simulink model "Simulation_Series"  (R2025b)
settings: Solver=VariableStepAuto  StartTime=0.0  StopTime=30000  RelTol=1e-6  EnableMultiTasking=on
PreLoadFcn:
  | % 1. Get the absolute path of the folder where this Simulink model is saved
  | model_dir = fileparts(get_param(bdroot, 'FileName'));
  | 
  | % 2. Add that folder and all subfolders (optimization, gp_models) to the MATLAB path
  | addpath(genpath(model_dir));
  | 
  | % 3. Print a success message to the Command Window so the user knows it worked
  | disp(['[RTO Setup] Successfully loaded paths for model: ', bdroot]);
InitFcn:
  | X_init_series
values from neighbouring files (symbols this model uses):
  Xinit1 = [          95322.9245471678 ... (first row only)    [X_init_series.m]
  Xinit2 = [139339.471687902 ... (first row only)    [X_init_series.m]
libraries: slpidlib x2, simulink x1
settings Model: Creator=chmemer  LastModifiedBy=ld719
settings SolverCC: AlgebraicLoopSolver=TrustRegion
settings DataIOCC: LimitDataPoints=on  SaveFinalState=on  SaveFormat=Array  SignalLoggingSaveFormat=ModelDataLogs  ReturnWorkspaceOutputs=off
settings OptimizationCC: ExpressionDepthLimit=2147483647.0  LifeSpan=inf
settings DebuggingCC: UnderspecifiedInitializationDetection=Classic  MergeDetectMultiDrivingBlocksExec=none  SolverPrmCheckMsg=warning  FcnCallInpInsideContextMsg=warning  UnconnectedInputMsg=warning  UnconnectedOutputMsg=warning  UnconnectedLineMsg=warning  StateNameClashWarn=warning  SFUnexpectedBacktrackingDiag=warning  SFNoUnconditionalDefaultTransitionDiag=warning  SFExecutionAtInitializationDiag=none  ArithmeticOperatorsInVariantConditions=warning
settings HardwareCC: ProdBitPerPointer=32.0  ProdBitPerSizeT=32.0  ProdBitPerPtrDiffT=32.0  ProdLargestAtomicFloat=None  ProdIntDivRoundTo=Undefined  ProdEndianess=Unspecified  ProdWordSize=32.0  ProdHWDeviceType=32-bit Generic
settings ModelReferenceCC: EnableRefExpFcnMdlSchedulingChecks=on  PropagateSignalLabelsOutOfModel=off
settings SFSimCC: SimUseLocalCustomCode=off  CustomCodeUndefinedFunction=UseInterfaceOnly
settings RTWCC: RTWUseLocalCustomCode=off  GPUComputeCapability=3.5
settings CodeAppCC: StateflowObjectComments=on
settings GRTTargetCC: TargetLangStandard=C89/C90 (ANSI)  CombineOutputUpdateFcns=off  GRTInterface=on
settings ConfigComp: CovMetricSettings=dw  CovSaveCumulativeToWorkspaceVar=on  CovSaveSingleToWorkspaceVar=on  CovExternalEMLEnable=off  CovSFcnEnable=off

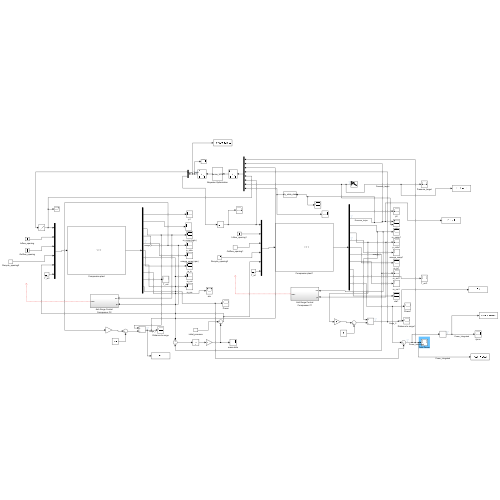
[thumbnail: Simulink's stored preview of the top-level diagram]
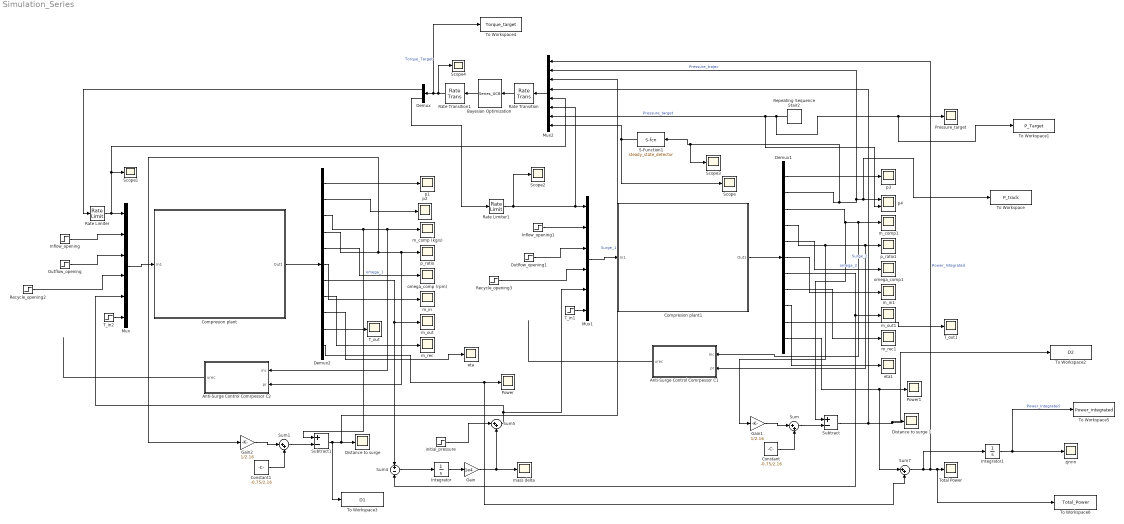
== system Simulation_Series ==
  Anti-Surge Control Comrpessor C1 : Subsystem
  Anti-Surge Control Comrpessor C2 : Subsystem
  Bayesian Optimization : S-Function  FunctionName=Series_UCB  SFunctionDeploymentMode=off  EnableBusSupport=off
  Compresion plant : Subsystem
      mask Display: image(imread('comp_plant.jpg'))
  Compresion plant1 : Subsystem
      mask Display: image(imread('comp_plant.jpg'))
  Constant : Constant  Value=-0.75/2.16
  Constant1 : Constant  Value=-0.75/2.16
  Demux : Demux  Outputs=2
  Demux1 : Demux  Outputs=11
  Demux2 : Demux  Outputs=11
  Distance to surge : Scope
      settings: ActiveDisplayYMinimum=0.077548735618170245  ActiveDisplayYMaximum=0.26199999787444433  DataLoggingVariableName=ScopeData2
  Distance to surge 1 : Scope
      settings: ActiveDisplayYMinimum=-0.020292289353042135  ActiveDisplayYMaximum=0.33961238201814714
  Gain : Gain  Gain=1e4
  Gain1 : Gain  Gain=1/2.16
  Gain2 : Gain  Gain=1/2.16
  Inflow_opening : Step  Time=25  Before=0.5  After=0.5  SampleTime=0
  Inflow_opening1 : Step  Time=25  Before=0.4541  After=0.4541  SampleTime=0
  Integrator : Integrator
  Integrator1 : Integrator
  Mux : Mux  Inputs=6
  Mux1 : Mux  Inputs=6
  Mux2 : Mux  Inputs=8
  Outflow_opening : Step  Time=10  Before=0.46  After=0.46  SampleTime=0
  Outflow_opening1 : Step  Time=10  Before=0.56  After=0.56  SampleTime=0
  Power : Scope
      settings: ActiveDisplayYMinimum=100000  ActiveDisplayYMaximum=300000  DataLoggingVariableName=ScopeData3  DataLoggingSaveFormat=Array
  Power1 : Scope
      settings: ActiveDisplayYMinimum=30000  ActiveDisplayYMaximum=70000  DataLoggingVariableName=ScopeData4  DataLoggingSaveFormat=Array
  Pressure_target : Scope
      settings: ActiveDisplayYMinimum=-1  ActiveDisplayYMaximum=1  DataLoggingVariableName=ScopeData5
  Rate Limiter : RateLimiter  RisingSlewLimit=0.1  FallingSlewLimit=-0.1  SampleTimeMode=inherited
  Rate Limiter1 : RateLimiter  RisingSlewLimit=0.1  FallingSlewLimit=-0.1  SampleTimeMode=inherited
  Rate Transition : RateTransition
  Rate Transition1 : RateTransition  InitialCondition=[20;20]
  Recycle_opening2 : Step  Time=2.05  After=0  SampleTime=0
  Recycle_opening3 : Step  Time=2.05  After=0  SampleTime=0
  Repeating Sequence Stair2 : simulink/Sources/Repeating Sequence Stair  OutValues=[248000 244000 246000 243000 242000 241000].'  tsamp=5000  OutMin=[]  OutMax=[]  OutDataTypeStr=double  OutputDataTypeScalingMode=double  OutDataType=fixdt(0,8)  ConRadixGroup=Best Precision: Vector-wise  OutScaling=2^-12
  S-Function1 : S-Function  FunctionName=steady_state_detector  SFunctionDeploymentMode=off  EnableBusSupport=off
  Scope{,1..4} (5 alike) : Scope
      Scope settings: ActiveDisplayYMinimum=-0.12499999999999997  ActiveDisplayYMaximum=1.125
      Scope1 settings: ActiveDisplayYMinimum=12.704969172625178  ActiveDisplayYMaximum=20.810558980819426  DataLoggingVariableName=ScopeData2
      Scope2 settings: ActiveDisplayYMinimum=14.056047000321247  ActiveDisplayYMaximum=20.660439222186529  DataLoggingVariableName=ScopeData3
      Scope3 settings: ActiveDisplayYMinimum=240000  ActiveDisplayYMaximum=250000
      Scope4 settings: ActiveDisplayYMinimum=10.651075634209118  ActiveDisplayYMaximum=21.457913073387115
  Subtract : Sum  Inputs=+-
  Subtract1 : Sum  Inputs=+-
  Sum{,1,5,7} (4 alike) : Sum  Inputs=|++
  Sum4 : Sum  Inputs=+|-
  T_in1 : Step  Time=2  Before=273+20  After=273+20  SampleTime=0
  T_in2 : Step  Time=2  Before=273+20  After=273+20  SampleTime=0
  T_out : Scope
      settings: ActiveDisplayYMinimum=-1  ActiveDisplayYMaximum=1
  T_out1 : Scope
      settings: ActiveDisplayYMinimum=97544.29295  ActiveDisplayYMaximum=97745.86123  DataLoggingVariableName=ScopeData2
  To Workspace : ToWorkspace  VariableName=P_track  SaveFormat=Structure With Time  SampleTime=1
  To Workspace1 : ToWorkspace  VariableName=P_Target  SaveFormat=Structure With Time  SampleTime=1
  To Workspace2 : ToWorkspace  VariableName=D2  SaveFormat=Structure With Time  SampleTime=1
  To Workspace3 : ToWorkspace  VariableName=D1  SaveFormat=Structure With Time  SampleTime=1
  To Workspace4 : ToWorkspace  VariableName=Torque_target  SaveFormat=Structure With Time  SampleTime=1
  To Workspace5 : ToWorkspace  VariableName=Power_integrated  SaveFormat=Structure With Time  SampleTime=1
  To Workspace6 : ToWorkspace  VariableName=Total_Power  SaveFormat=Structure With Time  SampleTime=1
  Total Power : Scope
      settings: ActiveDisplayYMinimum=87673.50775599209  ActiveDisplayYMaximum=243371.1571212415  DataLoggingVariableName=ScopeData3
  eta : Scope
      settings: ActiveDisplayYMinimum=0.21745085276170312  ActiveDisplayYMaximum=0.23352090021491981  DataLoggingSaveFormat=Array
  eta1 : Scope
      settings: ActiveDisplayYMinimum=0.84842072953292291  ActiveDisplayYMaximum=0.8942963809934541  DataLoggingVariableName=ScopeData2  DataLoggingSaveFormat=Array
  initial_pressure : Step  Time=30  Before=148276.78289724  After=148276.78289724  SampleTime=0
  m_comp (kg/s) : Scope
      settings: ActiveDisplayYMinimum=0.40770202444342352  ActiveDisplayYMaximum=0.84430507901595309  DataLoggingVariableName=m_comp  DataLoggingSaveFormat=Array
  m_comp1 : Scope
      settings: ActiveDisplayYMinimum=0.60292  ActiveDisplayYMaximum=0.60459  DataLoggingVariableName=m_comp1  DataLoggingSaveFormat=Array
  m_in : Scope
      settings: ActiveDisplayYMinimum=0.60226  ActiveDisplayYMaximum=0.61057  DataLoggingVariableName=ScopeData2
  m_in1 : Scope
      settings: DataLoggingVariableName=ScopeData11
  m_out : Scope
      settings: ActiveDisplayYMinimum=0.42270198893071659  ActiveDisplayYMaximum=0.77722336304535555  DataLoggingVariableName=ScopeData3
  m_out1 : Scope
      settings: ActiveDisplayYMinimum=0.50120300179820743  ActiveDisplayYMaximum=0.71721824106829912  DataLoggingVariableName=ScopeData13
  m_rec : Scope
      settings: ActiveDisplayYMinimum=-1  ActiveDisplayYMaximum=1  DataLoggingVariableName=m_rec  DataLoggingSaveFormat=Array
  m_rec1 : Scope
      settings: ActiveDisplayYMinimum=-1  ActiveDisplayYMaximum=1  DataLoggingVariableName=m_rec1  DataLoggingSaveFormat=Array
  mass delta : Scope
      settings: ActiveDisplayYMinimum=-1573.08764  ActiveDisplayYMaximum=14157.77212
  omega_comp (rpm) : Scope
      settings: TimeSpan=10  ActiveDisplayYMinimum=3418.211911212803  ActiveDisplayYMaximum=3418.2119165301274  DataLoggingVariableName=ScopeData4
  omega_comp1 : Scope
      settings: TimeSpan=10  ActiveDisplayYMinimum=3403.3405459456822  ActiveDisplayYMaximum=4015.4960771962442  DataLoggingVariableName=ScopeData14
  p1 : Scope
      settings: ActiveDisplayYMinimum=96759.18199  ActiveDisplayYMaximum=106424.4061
  p2 : Scope
      settings: TimeSpan=800  ActiveDisplayYMinimum=142686.83533455073  ActiveDisplayYMaximum=177417.85344844157
  p3 : Scope
      settings: ActiveDisplayYMinimum=129412.56133  ActiveDisplayYMaximum=141037.29748  DataLoggingVariableName=ScopeData15
  p4 : Scope  NumInputPorts=2
      settings: TimeSpan=16000  ActiveDisplayYMinimum=240988.04397616221  ActiveDisplayYMaximum=249610.22414713461  DataLoggingVariableName=ScopeData16
  p_ratio : Scope
      settings: ActiveDisplayYMinimum=1.4510137511633545  ActiveDisplayYMaximum=1.8639764896836617  DataLoggingVariableName=p_ratio  DataLoggingSaveFormat=Array
  p_ratio1 : Scope
      settings: ActiveDisplayYMinimum=1.7222858302327289  ActiveDisplayYMaximum=2.0157667356513191  DataLoggingVariableName=p_ratio1  DataLoggingSaveFormat=Array
  zjnnn : Scope
      settings: ActiveDisplayYMinimum=-2.475946022057547E+8  ActiveDisplayYMaximum=2.2283514198517928E+9
  wires:
  Compresion plant/1(Out1) -> Demux2/1
  Mux/1 -> Compresion plant/1(In1)
  Demux2/3 -> Anti-Surge Control Comrpessor C2/1(mc), m_comp (kg/s)/1, Subtract1/1
  Demux2/4 -> Gain2/1, p_ratio/1, Anti-Surge Control Comrpessor C2/2(pr)
  Demux2/5 -> omega_comp (rpm)/1  "omega_1"
  Outflow_opening/1 -> Mux/3
  Anti-Surge Control Comrpessor C2/1(urec) -> ?
  Demux2/6 -> m_in/1
  Demux2/1 -> p1/1
  Demux2/2 -> p2/1
  Demux2/8 -> m_rec/1
  Demux1/8 -> m_rec1/1
  Demux1/1 -> p3/1
  Demux1/7 -> Sum4/2, m_out1/1
  Demux1/6 -> m_in1/1
  Anti-Surge Control Comrpessor C1/1(urec) -> ?
  Outflow_opening1/1 -> Mux1/3
  Demux1/5 -> omega_comp1/1  "omega_2"
  Demux1/4 -> Gain1/1, Anti-Surge Control Comrpessor C1/2(pr), p_ratio1/1
  Demux1/3 -> Subtract/1, Anti-Surge Control Comrpessor C1/1(mc), m_comp1/1
  Mux1/1 -> Compresion plant1/1(In1)
  Compresion plant1/1(Out1) -> Demux1/1
  Sum4/1 -> Integrator/1
  Integrator/1 -> Gain/1
  initial_pressure/1 -> Sum5/1
  Sum5/1 -> Mux/5, Mux1/5
  Gain/1 -> Sum5/2, mass delta/1
  Demux2/9 -> eta/1
  Demux2/11 -> Sum7/2, Power/1
  Demux2/10 -> T_out/1
  Inflow_opening/1 -> Mux/2
  Demux1/9 -> eta1/1
  Demux1/11 -> Sum7/1, Power1/1
  T_in2/1 -> Mux/6
  Inflow_opening1/1 -> Mux1/2
  T_in1/1 -> Mux1/6
  Demux1/10 -> T_out1/1
  Integrator1/1 -> To Workspace5/1, zjnnn/1  "Power_Integrated"
  Demux2/7 -> m_out/1, Sum4/1
  Gain1/1 -> Sum/1
  Constant/1 -> Sum/2
  Sum/1 -> Subtract/2
  Subtract/1 -> Mux2/4, To Workspace2/1, Distance to surge 1/1  "Surge_2"
  Constant1/1 -> Sum1/2
  Sum1/1 -> Subtract1/2
  Gain2/1 -> Sum1/1
  Subtract1/1 -> Distance to surge/1, Mux2/3, To Workspace3/1  "Surge_1"
  Repeating Sequence Stair2/1 -> To Workspace1/1, Pressure_target/1, p4/2, Mux2/7  "Pressure_target"
  S-Function1/1 -> Mux2/8, Scope/1
  Mux2/1 -> Rate Transition/1
  Bayesian Optimization/1 -> Rate Transition1/1
  Demux1/2 -> Scope3/1, S-Function1/1, Mux2/2, To Workspace/1, p4/1  "Pressure_trajec"
  Rate Limiter1/1 -> Scope2/1, Mux2/6, Mux1/1
  Rate Limiter/1 -> Scope1/1, Mux2/5, Mux/1
  Rate Transition/1 -> Bayesian Optimization/1
  Rate Transition1/1 -> Scope4/1, To Workspace4/1, Demux/1  "Torque_Target"
  Demux/2 -> Rate Limiter1/1
  Demux/1 -> Rate Limiter/1
  Sum7/1 -> Integrator1/1, To Workspace6/1, Total Power/1, Mux2/1  "Power_Integrated"
  Recycle_opening2/1 -> Mux/4
  Recycle_opening3/1 -> Mux1/4

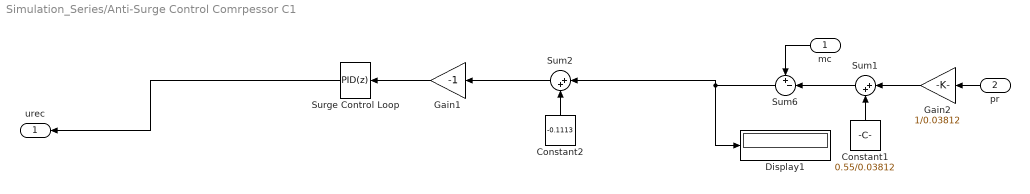
== system Simulation_Series/Anti-Surge Control Comrpessor C1 ==
  mc : Inport
  pr : Inport  Port=2
  Constant1 : Constant  Value=0.55/0.03812
  Constant2 : Constant  Value=-0.1113
  Display1 : Display
  Gain1 : Gain  Gain=-1
  Gain2 : Gain  Gain=1/0.03812
  Sum1 : Sum  Inputs=|++
  Sum2 : Sum  Inputs=|++
  Sum6 : Sum  Inputs=+-|
  Surge Control Loop : slpidlib/PID Controller  Controller=PID  Form=Parallel  TimeDomain=Discrete-time  UseExternalTs=off  SampleTime=0.5  IntegratorMethod=Forward Euler  FilterMethod=Forward Euler  ControllerParametersSource=internal  P=0.05  I=0.01  UseKiTs=off  D=0  UseExternalDerivativeSource=off  N=2.82959055969234  UseFilter=on  TunerSelectOption=Transfer Function Based (PID Tuner App)  ZeroCross=off  InitialConditionSource=internal  InitialConditionForIntegrator=0  InitialConditionForFilter=0  DifferentiatorICPrevScaledInput=0  ExternalReset=none  TrackingMode=off  Kt=1  LimitOutput=on  SatLimitsSource=internal  UpperSaturationLimit=1  LowerSaturationLimit=0  LinearizeAsGain=off  AntiWindupMode=back-calculation  Kb=1  LimitIntegrator=off  UpperIntegratorSaturationLimit=inf  LowerIntegratorSaturationLimit=-inf  POutMin=[]  POutMax=[]  IOutMin=[]  IOutMax=[]  DOutMin=[]  DOutMax=[]  NOutMin=[]  NOutMax=[]  SumOutMin=[]  SumOutMax=[]  SaturationOutMin=[]  SaturationOutMax=[]  PParamMin=[]  PParamMax=[]  IParamMin=[]  IParamMax=[]  DParamMin=[]  DParamMax=[]  NParamMin=[]  NParamMax=[]  KbParamMin=[]  KbParamMax=[]  KtParamMin=[]  KtParamMax=[]  KbOutMin=[]  KbOutMax=[]  KtOutMin=[]  KtOutMax=[]  IntegratorOutMin=[]  IntegratorOutMax=[]  FilterOutMin=[]  FilterOutMax=[]  SumI1OutMin=[]  SumI1OutMax=[]  SumI2OutMin=[]  SumI2OutMax=[]  SumI3OutMin=[]  SumI3OutMax=[]  SumI4OutMin=[]  SumI4OutMax=[]  SumDOutMin=[]  SumDOutMax=[]  DifferentiatorOutMin=[]  DifferentiatorOutMax=[]  FilterDiffOutCoefMin=[]  FilterDiffOutCoefMax=[]  ReciprocalOutMin=[]  ReciprocalOutMax=[]  SumDenOutMin=[]  SumDenOutMax=[]  SumNumOutMin=[]  SumNumOutMax=[]  DivideOutMin=[]  DivideOutMax=[]  UdiffTsProdOutMin=[]  UdiffTsProdOutMax=[]  NTsProdOutMin=[]  NTsProdOutMax=[]  UintegralTsProdOutMin=[]  UintegralTsProdOutMax=[]  UngainTsProdOutMin=[]  UngainTsProdOutMax=[]  ClampingZeroOutDataTypeStr=Inherit: Inherit via back propagation  ClampingZeroOutMin=[]  ClampingZeroOutMax=[]  FilterDenConstantOutDataTypeStr=Inherit: Inherit via back propagation  FilterDenConstantOutMin=[]  FilterDenConstantOutMax=[]  PCopyOutDataTypeStr=Inherit: Inherit via back propagation  PCopyOutMin=[]  PCopyOutMax=[]  NCopyOutDataTypeStr=Inherit: Inherit via back propagation  NCopyOutMin=[]  NCopyOutMax=[]  IntegratorContinuousStateAttributes=''  IntegratorStateMustResolveToSignalObject=off  IntegratorRTWStateStorageClass=Auto  FilterContinuousStateAttributes=''  FilterStateMustResolveToSignalObject=off  FilterRTWStateStorageClass=Auto  ParallelPVariant=InternalParameters  IdealPVariant=Disabled  IVariant=InternalParameters  DVariant=InternalParameters  IntegratorVariant=Discrete  SatVariant=Enabled  AWVariant=BackCalculation  PCopyVariant=Disabled  TRVariant=Disabled  FdbkBlocksVariant=Forward  IdealPFdbkVariant=Disabled  SatFdbkVariant=Disabled  DerivativeFilterVariant=ForwardEulerFilter  NVariant=InternalParameters  NCopyVariant=Disabled  FilterICVariant=InternalICsFilter  IntegratorICVariant=InternalICs  ExternalResetVariant=Disabled  TRSumVariant=Passthrough  SumFdbkVariant=Disabled  SumVariant=Sum_PID  TsampFilterVariant=InternalTs  TsampNgainVariant=Passthrough  TsampIntegralVariant=Disabled_SignalSpec  ExternalSaturationOutDataTypeStr=Inherit: Same as second input  DerivativeSourceVariant=ErrorSignal  PreIntVariant=InternalPreInt
  urec : Outport
  wires:
  Gain2/1 -> Sum1/1
  Constant1/1 -> Sum1/2
  Sum1/1 -> Sum6/2
  Sum6/1 -> Sum2/1, Display1/1
  Surge Control Loop/1 -> urec/1
  mc/1 -> Sum6/1
  pr/1 -> Gain2/1
  Gain1/1 -> Surge Control Loop/1
  Sum2/1 -> Gain1/1
  Constant2/1 -> Sum2/2

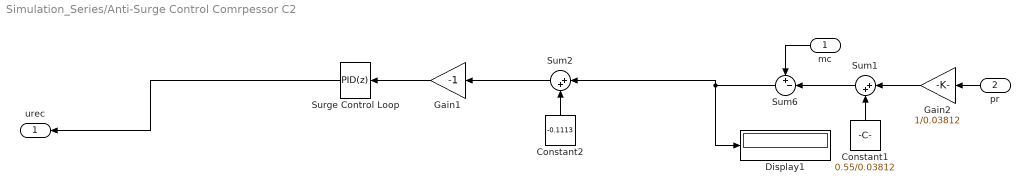
== system Simulation_Series/Anti-Surge Control Comrpessor C2 ==
  mc : Inport
  pr : Inport  Port=2
  Constant1 : Constant  Value=0.55/0.03812
  Constant2 : Constant  Value=-0.1113
  Display1 : Display
  Gain1 : Gain  Gain=-1
  Gain2 : Gain  Gain=1/0.03812
  Sum1 : Sum  Inputs=|++
  Sum2 : Sum  Inputs=|++
  Sum6 : Sum  Inputs=+-|
  Surge Control Loop : slpidlib/PID Controller  Controller=PID  Form=Parallel  TimeDomain=Discrete-time  UseExternalTs=off  SampleTime=0.5  IntegratorMethod=Forward Euler  FilterMethod=Forward Euler  ControllerParametersSource=internal  P=0.05  I=0.01  UseKiTs=off  D=0  UseExternalDerivativeSource=off  N=2.82959055969234  UseFilter=on  TunerSelectOption=Transfer Function Based (PID Tuner App)  ZeroCross=off  InitialConditionSource=internal  InitialConditionForIntegrator=0  InitialConditionForFilter=0  DifferentiatorICPrevScaledInput=0  ExternalReset=none  TrackingMode=off  Kt=1  LimitOutput=on  SatLimitsSource=internal  UpperSaturationLimit=1  LowerSaturationLimit=0  LinearizeAsGain=off  AntiWindupMode=back-calculation  Kb=1  LimitIntegrator=off  UpperIntegratorSaturationLimit=inf  LowerIntegratorSaturationLimit=-inf  POutMin=[]  POutMax=[]  IOutMin=[]  IOutMax=[]  DOutMin=[]  DOutMax=[]  NOutMin=[]  NOutMax=[]  SumOutMin=[]  SumOutMax=[]  SaturationOutMin=[]  SaturationOutMax=[]  PParamMin=[]  PParamMax=[]  IParamMin=[]  IParamMax=[]  DParamMin=[]  DParamMax=[]  NParamMin=[]  NParamMax=[]  KbParamMin=[]  KbParamMax=[]  KtParamMin=[]  KtParamMax=[]  KbOutMin=[]  KbOutMax=[]  KtOutMin=[]  KtOutMax=[]  IntegratorOutMin=[]  IntegratorOutMax=[]  FilterOutMin=[]  FilterOutMax=[]  SumI1OutMin=[]  SumI1OutMax=[]  SumI2OutMin=[]  SumI2OutMax=[]  SumI3OutMin=[]  SumI3OutMax=[]  SumI4OutMin=[]  SumI4OutMax=[]  SumDOutMin=[]  SumDOutMax=[]  DifferentiatorOutMin=[]  DifferentiatorOutMax=[]  FilterDiffOutCoefMin=[]  FilterDiffOutCoefMax=[]  ReciprocalOutMin=[]  ReciprocalOutMax=[]  SumDenOutMin=[]  SumDenOutMax=[]  SumNumOutMin=[]  SumNumOutMax=[]  DivideOutMin=[]  DivideOutMax=[]  UdiffTsProdOutMin=[]  UdiffTsProdOutMax=[]  NTsProdOutMin=[]  NTsProdOutMax=[]  UintegralTsProdOutMin=[]  UintegralTsProdOutMax=[]  UngainTsProdOutMin=[]  UngainTsProdOutMax=[]  ClampingZeroOutDataTypeStr=Inherit: Inherit via back propagation  ClampingZeroOutMin=[]  ClampingZeroOutMax=[]  FilterDenConstantOutDataTypeStr=Inherit: Inherit via back propagation  FilterDenConstantOutMin=[]  FilterDenConstantOutMax=[]  PCopyOutDataTypeStr=Inherit: Inherit via back propagation  PCopyOutMin=[]  PCopyOutMax=[]  NCopyOutDataTypeStr=Inherit: Inherit via back propagation  NCopyOutMin=[]  NCopyOutMax=[]  IntegratorContinuousStateAttributes=''  IntegratorStateMustResolveToSignalObject=off  IntegratorRTWStateStorageClass=Auto  FilterContinuousStateAttributes=''  FilterStateMustResolveToSignalObject=off  FilterRTWStateStorageClass=Auto  ParallelPVariant=InternalParameters  IdealPVariant=Disabled  IVariant=InternalParameters  DVariant=InternalParameters  IntegratorVariant=Discrete  SatVariant=Enabled  AWVariant=BackCalculation  PCopyVariant=Disabled  TRVariant=Disabled  FdbkBlocksVariant=Forward  IdealPFdbkVariant=Disabled  SatFdbkVariant=Disabled  DerivativeFilterVariant=ForwardEulerFilter  NVariant=InternalParameters  NCopyVariant=Disabled  FilterICVariant=InternalICsFilter  IntegratorICVariant=InternalICs  ExternalResetVariant=Disabled  TRSumVariant=Passthrough  SumFdbkVariant=Disabled  SumVariant=Sum_PID  TsampFilterVariant=InternalTs  TsampNgainVariant=Passthrough  TsampIntegralVariant=Disabled_SignalSpec  ExternalSaturationOutDataTypeStr=Inherit: Same as second input  DerivativeSourceVariant=ErrorSignal  PreIntVariant=InternalPreInt
  urec : Outport
  wires:
  Gain2/1 -> Sum1/1
  Constant1/1 -> Sum1/2
  Sum1/1 -> Sum6/2
  Sum6/1 -> Sum2/1, Display1/1
  Surge Control Loop/1 -> urec/1
  mc/1 -> Sum6/1
  pr/1 -> Gain2/1
  Gain1/1 -> Surge Control Loop/1
  Sum2/1 -> Gain1/1
  Constant2/1 -> Sum2/2

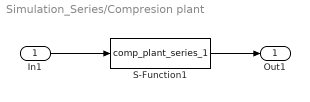
== system Simulation_Series/Compresion plant ==
  In1 : Inport
  S-Function1 : S-Function  FunctionName=comp_plant_series_1  Parameters=[], Xinit1  SFunctionDeploymentMode=off  EnableBusSupport=off
  Out1 : Outport  VectorParamsAs1DForOutWhenUnconnected=off
  wires:
  S-Function1/1 -> Out1/1
  In1/1 -> S-Function1/1

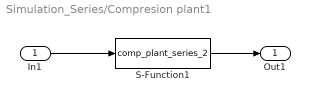
== system Simulation_Series/Compresion plant1 ==
  In1 : Inport
  S-Function1 : S-Function  FunctionName=comp_plant_series_2  Parameters=[], Xinit2  SFunctionDeploymentMode=off  EnableBusSupport=off
  Out1 : Outport  VectorParamsAs1DForOutWhenUnconnected=off
  wires:
  In1/1 -> S-Function1/1
  S-Function1/1 -> Out1/1
